simulink library "Meldas_library"  (R2016a)
settings: Solver=VariableStepAuto  SolverMode=SingleTasking  StartTime=0.0  StopTime=10.0  RelTol=1e-3
undefined symbols (not defined in the file): Cf, Iz, lf, m
settings Model: Creator=mulusoy  LastModifiedBy=thuha
settings DebuggingCC: SFUnexpectedBacktrackingDiag=error  SFNoUnconditionalDefaultTransitionDiag=error
settings GRTTargetCC: TargetLangStandard=C99 (ISO)  GeneratePreprocessorConditionals=Use local settings
settings ConfigComp: CovMetricSettings=dwe  CovHtmlReporting=off  CovSaveCumulativeToWorkspaceVar=off  CovSaveSingleToWorkspaceVar=off  CovExternalEMLEnable=on

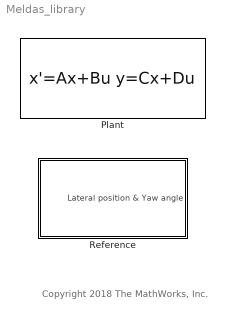
== system Meldas_library ==
  note: Copyright 2018 The MathWorks, Inc.
  Plant : StateSpace  A=|  B=[2*Cf/m 0 2*Cf*lf/Iz 0]';  C=[0 0 0 1; 0 1 0 0];  D=[0;0]  X0=0  mask{Vx=15}
      | [-(2*Cf+2*Cr)/m/Vx, 0, -Vx-(2*Cf*lf-2*Cr*lr)/m/Vx, 0;
      |      0, 0, 1, 0;
      |      -(2*Cf*lf-2*Cr*lr)/Iz/Vx, 0, -(2*Cf*lf^2+2*Cr*lr^2)/Iz/Vx, 0;
      |      1, Vx, 0, 0];
      mask Display: image("Car.jpg")
  Reference : Subsystem
      mask Display: image("Reference.jpg");

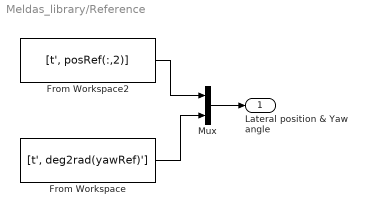
== system Meldas_library/Reference ==
  From Workspace : FromWorkspace  VariableName=[t', deg2rad(yawRef)']  SampleTime=0.1
  From Workspace2 : FromWorkspace  VariableName=[t', posRef(:,2)]  SampleTime=0.1
  Mux : Mux  Inputs=2
  Lateral position & Yaw angle : Outport
  wires:
  Mux/1 -> Lateral position & Yaw angle/1
  From Workspace/1 -> Mux/2
  From Workspace2/1 -> Mux/1
